simulink model "algebraic_loop_example"  (R2015a)
settings: Solver=ode4  StartTime=0.0  StopTime=10.0  FixedStep=0.01  RelTol=1e-3
libraries: simulink x3
settings Model: Creator=PD Banneheka  LastModifiedBy=PD Banneheka

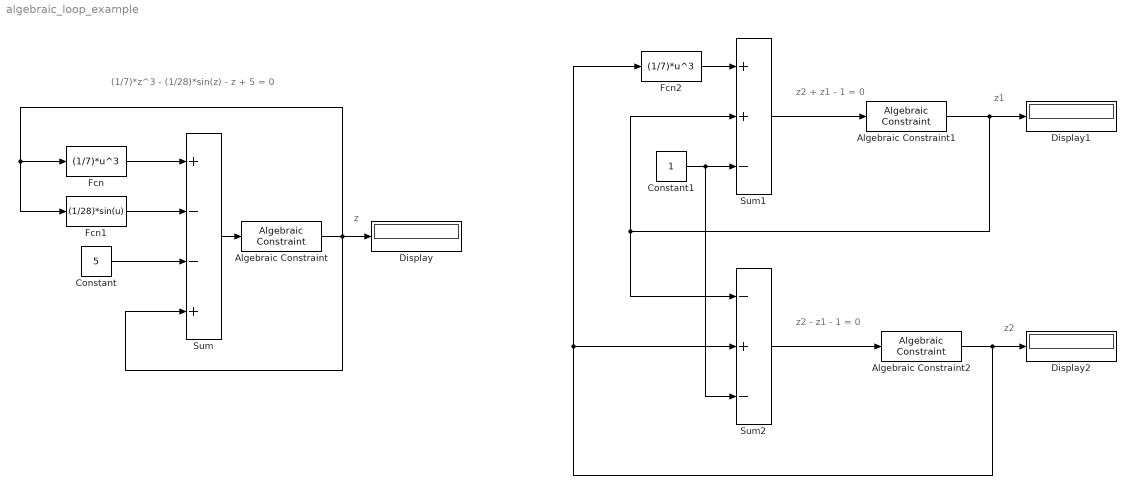
== system algebraic_loop_example ==
  note: z
  note: (1/7)*z^3 - (1/28)*sin(z) - z + 5 = 0
  note: z1
  note: z2 + z1 - 1 = 0
  note: z2
  note: z2 - z1 - 1 = 0
  Algebraic Constraint : simulink/Math Operations/Algebraic Constraint  z0=0
  Algebraic Constraint1 : simulink/Math Operations/Algebraic Constraint  z0=0
  Algebraic Constraint2 : simulink/Math Operations/Algebraic Constraint  z0=0
  Constant : Constant  Value=5
  Constant1 : Constant
  Display : Display
  Display1 : Display
  Display2 : Display
  Fcn : Fcn  Expr=(1/7)*u^3
  Fcn1 : Fcn  Expr=(1/28)*sin(u)
  Fcn2 : Fcn  Expr=(1/7)*u^3
  Sum : Sum  Inputs=+--+
  Sum1 : Sum  Inputs=++-
  Sum2 : Sum  Inputs=-+-
  wires:
  Fcn/1 -> Sum/1
  Fcn1/1 -> Sum/2
  Constant/1 -> Sum/3
  Sum/1 -> Algebraic Constraint/1
  Algebraic Constraint2/1 -> Display2/1, Sum2/2, Fcn2/1
  Sum1/1 -> Algebraic Constraint1/1
  Constant1/1 -> Sum2/3, Sum1/3
  Sum2/1 -> Algebraic Constraint2/1
  Algebraic Constraint1/1 -> Display1/1, Sum1/2, Sum2/1
  Algebraic Constraint/1 -> Sum/4, Fcn/1, Fcn1/1, Display/1
  Fcn2/1 -> Sum1/1
